simulink model "Factorial"  (R2025b)
settings: Solver=FixedStepDiscrete  StartTime=0.0  StopTime=10.0  FixedStep=0.01  RelTol=1e-3
settings Model: Creator=soura  LastModifiedBy=soura

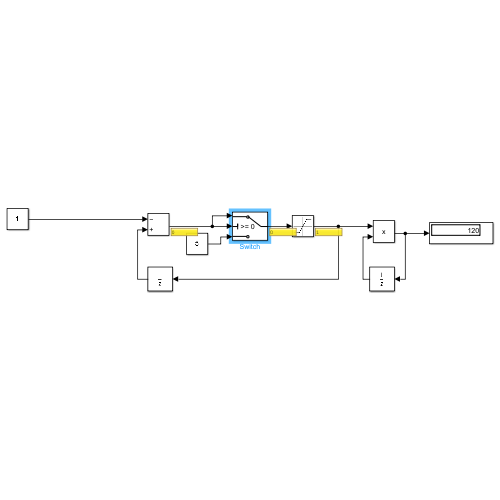
[thumbnail: Simulink's stored preview of the top-level diagram]
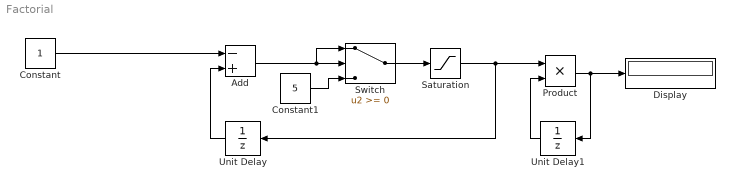
== system Factorial ==
  Add : Sum  Inputs=-+
  Constant : Constant
  Constant1 : Constant  Value=5
  Display : Display
  Product : Product
  Saturation : Saturate  UpperLimit=5  LowerLimit=1
  Switch : Switch  SaturateOnIntegerOverflow=off  InputSameDT=off
  Unit Delay : UnitDelay  SampleTime=-1  HasFrameUpgradeWarning=on
  Unit Delay1 : UnitDelay  InitialCondition=1  SampleTime=-1  HasFrameUpgradeWarning=on
  wires:
  Constant/1 -> Add/1
  Product/1 -> Display/1, Unit Delay1/1
  Unit Delay1/1 -> Product/2
  Add/1 -> Switch/1, Switch/2
  Switch/1 -> Saturation/1
  Unit Delay/1 -> Add/2
  Constant1/1 -> Switch/3
  Saturation/1 -> Unit Delay/1, Product/1
